simulink model "quantizedNetSim_4"  (R2025a)
settings: Solver=FixedStepAuto  StartTime=0.0  StopTime=10.0  RelTol=1e-3
undefined symbols (not defined in the file or in its folder): quantizedNet
libraries: dlconvfclib x9, dlactivationlib x3, dlpoolinglib x1, dlinputlayernormlib x1
settings Model: Creator=wenzheli  LastModifiedBy=wenzheli
settings OptimizationCC: DefaultParameterBehavior=Inlined  EnhancedBackFolding=on  PassReuseOutputArgsAs=Individual arguments  ZeroExternalMemoryAtStartup=off  ZeroInternalMemoryAtStartup=off  OptimizeBlockOrder=speed  DifferentSizesBufferReuse=on  OptimizationCustomize=off  EfficientTunableParamExpr=on
settings DebuggingCC: ParameterTunabilityLossMsg=error
settings SFSimCC: MATLABDynamicMemAlloc=off
settings RTWCC: SystemTargetFile=ert.tlc  TemplateMakefile=ert_default_tmf  Description=Embedded Coder
settings CodeAppCC: ForceParamTrailComments=on  IgnoreCustomStorageClasses=off  OperatorAnnotations=on  SimulinkDataObjDesc=on  SFDataObjDesc=on  InsertBlockDesc=on
settings ERTTargetCC: ExtModeTransport=0.0  ExtModeStaticAlloc=off  ExtModeMexFile=ext_comm  ExtModeIntrfLevel=Level1  ERTCustomFileTemplate=example_file_process.tlc  TargetLangStandard=C99 (ISO)  GenerateSampleERTMain=on

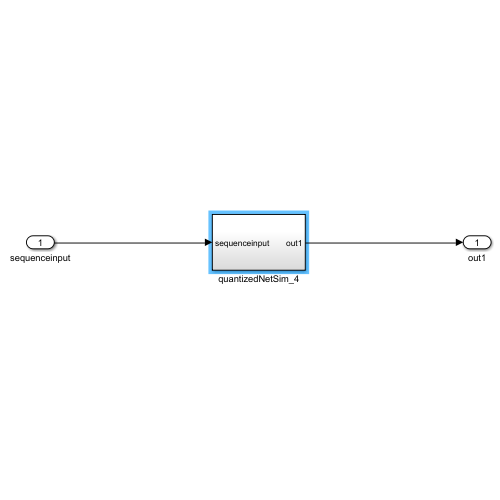
[thumbnail: Simulink's stored preview of the top-level diagram]
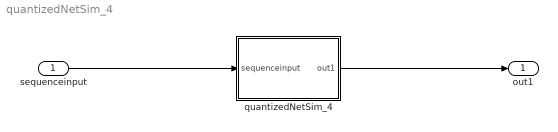
== system quantizedNetSim_4 ==
  sequenceinput : Inport  PortDimensions="[1  256]"
  quantizedNetSim_4 : Subsystem
  out1 : Outport
  wires:
  sequenceinput/1 -> quantizedNetSim_4/1(sequenceinput)
  quantizedNetSim_4/1(out1) -> out1/1

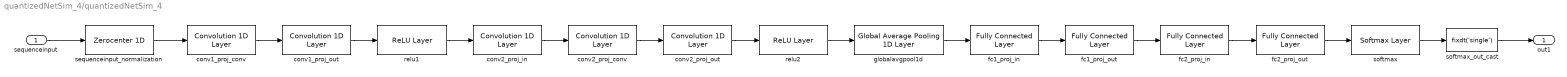
== system quantizedNetSim_4/quantizedNetSim_4 ==
  sequenceinput : Inport  PortDimensions="[1  256]"
  conv1_proj_conv : dlconvfclib/Convolution 1D Layer  Layer=quantizedNet.Layers(2)  PermuteDims=[2 1]  OutMin=[]  OutMax=[]  OutDataTypeStr=fixdt(1,8,1)  RndMeth=Nearest  SaturateOnIntegerOverflow=on  WeightsDataTypeStr=fixdt(1,8,7)  WeightsMin=[]  WeightsMax=[]  BiasDataTypeStr=fixdt(1,32,10)  BiasMin=[]  BiasMax=[]  AccumDataTypeStr=fixdt(1,32,10)  InternalRndMeth=Nearest  InternalSaturateOnIntegerOverflow=off  SampleTime=-1
      settings: DataFormat=CT
  conv1_proj_out : dlconvfclib/Convolution 1D Layer  Layer=quantizedNet.Layers(3)  PermuteDims=[2 1]  OutMin=[]  OutMax=[]  OutDataTypeStr=fixdt(1,8,2)  RndMeth=Nearest  SaturateOnIntegerOverflow=on  WeightsDataTypeStr=fixdt(1,8,7)  WeightsMin=[]  WeightsMax=[]  BiasDataTypeStr=fixdt(1,32,8)  BiasMin=[]  BiasMax=[]  AccumDataTypeStr=fixdt(1,32,8)  InternalRndMeth=Nearest  InternalSaturateOnIntegerOverflow=off  SampleTime=-1
      settings: DataFormat=CT
  conv2_proj_conv : dlconvfclib/Convolution 1D Layer  Layer=quantizedNet.Layers(6)  PermuteDims=[2 1]  OutMin=[]  OutMax=[]  OutDataTypeStr=fixdt(1,8,-2)  RndMeth=Nearest  SaturateOnIntegerOverflow=on  WeightsDataTypeStr=fixdt(1,8,7)  WeightsMin=[]  WeightsMax=[]  BiasDataTypeStr=fixdt(1,32,8)  BiasMin=[]  BiasMax=[]  AccumDataTypeStr=fixdt(1,32,8)  InternalRndMeth=Nearest  InternalSaturateOnIntegerOverflow=off  SampleTime=-1
      settings: DataFormat=CT
  conv2_proj_in : dlconvfclib/Convolution 1D Layer  Layer=quantizedNet.Layers(5)  PermuteDims=[2 1]  OutMin=[]  OutMax=[]  OutDataTypeStr=fixdt(1,8,1)  RndMeth=Nearest  SaturateOnIntegerOverflow=on  WeightsDataTypeStr=fixdt(1,8,7)  WeightsMin=[]  WeightsMax=[]  BiasDataTypeStr=fixdt(1,32,9)  BiasMin=[]  BiasMax=[]  AccumDataTypeStr=fixdt(1,32,9)  InternalRndMeth=Nearest  InternalSaturateOnIntegerOverflow=off  SampleTime=-1
      settings: DataFormat=CT
  conv2_proj_out : dlconvfclib/Convolution 1D Layer  Layer=quantizedNet.Layers(7)  PermuteDims=[2 1]  OutMin=[]  OutMax=[]  OutDataTypeStr=fixdt(1,8,-2)  RndMeth=Nearest  SaturateOnIntegerOverflow=on  WeightsDataTypeStr=fixdt(1,8,7)  WeightsMin=[]  WeightsMax=[]  BiasDataTypeStr=fixdt(1,32,5)  BiasMin=[]  BiasMax=[]  AccumDataTypeStr=fixdt(1,32,5)  InternalRndMeth=Nearest  InternalSaturateOnIntegerOverflow=off  SampleTime=-1
      settings: DataFormat=CT
  fc1_proj_in : dlconvfclib/Fully Connected Layer  Layer=quantizedNet.Layers(10)  OutMin=[]  OutMax=[]  OutDataTypeStr=fixdt(1,8,5)  RndMeth=Nearest  SaturateOnIntegerOverflow=on  WeightsDataTypeStr=fixdt(1,8,7)  WeightsMin=[]  WeightsMax=[]  BiasDataTypeStr=fixdt(1,32,10)  BiasMin=[]  BiasMax=[]  AccumDataTypeStr=fixdt(1,32,10)  AccumMin=[]  AccumMax=[]  InternalRndMeth=Nearest  InternalSaturateOnIntegerOverflow=off  SampleTime=-1
      settings: DataFormat=C
  fc1_proj_out : dlconvfclib/Fully Connected Layer  Layer=quantizedNet.Layers(11)  OutMin=[]  OutMax=[]  OutDataTypeStr=fixdt(1,8,6)  RndMeth=Nearest  SaturateOnIntegerOverflow=on  WeightsDataTypeStr=fixdt(1,8,7)  WeightsMin=[]  WeightsMax=[]  BiasDataTypeStr=fixdt(1,32,12)  BiasMin=[]  BiasMax=[]  AccumDataTypeStr=fixdt(1,32,12)  AccumMin=[]  AccumMax=[]  InternalRndMeth=Nearest  InternalSaturateOnIntegerOverflow=off  SampleTime=-1
      settings: DataFormat=C
  fc2_proj_in : dlconvfclib/Fully Connected Layer  Layer=quantizedNet.Layers(12)  OutMin=[]  OutMax=[]  OutDataTypeStr=fixdt(1,8,2)  RndMeth=Nearest  WeightsDataTypeStr=fixdt(1,8,7)  WeightsMin=[]  WeightsMax=[]  BiasDataTypeStr=fixdt(1,32,13)  BiasMin=[]  BiasMax=[]  AccumDataTypeStr=fixdt(1,32,13)  AccumMin=[]  AccumMax=[]  InternalRndMeth=Nearest  InternalSaturateOnIntegerOverflow=off  SampleTime=-1
      settings: DataFormat=C
  fc2_proj_out : dlconvfclib/Fully Connected Layer  Layer=quantizedNet.Layers(13)  OutMin=[]  OutMax=[]  OutDataTypeStr=fixdt(1,8,2)  RndMeth=Nearest  SaturateOnIntegerOverflow=on  WeightsDataTypeStr=fixdt(1,8,7)  WeightsMin=[]  WeightsMax=[]  BiasDataTypeStr=fixdt(1,32,9)  BiasMin=[]  BiasMax=[]  AccumDataTypeStr=fixdt(1,32,9)  AccumMin=[]  AccumMax=[]  InternalRndMeth=Nearest  InternalSaturateOnIntegerOverflow=off  SampleTime=-1
      settings: DataFormat=C
  globalavgpool1d : dlpoolinglib/Global Average Pooling 1D Layer  Layer=quantizedNet.Layers(9)  InputSize="[2  256]"  OutMin=[]  OutMax=[]  OutDataTypeStr=fixdt(1,8,3)  RndMeth=Nearest  SaturateOnIntegerOverflow=on  AccumDataTypeStr=fixdt(1,32,-2)  NumPoolingElementsDataTypeStr=fixdt(0,32,0)  NumPoolingElementsMin=[]  NumPoolingElementsMax=[]  InternalRndMeth=Nearest  InternalSaturateOnIntegerOverflow=on  SampleTime=-1
      settings: DataFormat=CT
  relu1 : dlactivationlib/ReLU Layer  OutMin=[]  OutMax=[]  OutDataTypeStr=fixdt(1,8,2)  SampleTime=-1
  relu2 : dlactivationlib/ReLU Layer  OutMin=[]  OutMax=[]  OutDataTypeStr=fixdt(1,8,-2)  SampleTime=-1
  sequenceinput_normalization : dlinputlayernormlib/Zerocenter 1D  Layer=quantizedNet.Layers(1)  OutMin=[]  OutMax=[]  OutDataTypeStr=fixdt(1,8,3)  RndMeth=Nearest  SaturateOnIntegerOverflow=on  MeanDataTypeStr=fixdt(0,8,13)  MeanMin=[]  MeanMax=[]  AccumDataTypeStr=fixdt(1,21,13)  InternalRndMeth=Nearest  InternalSaturateOnIntegerOverflow=on  SampleTime=-1
      settings: DataFormat=CT
  softmax : dlactivationlib/Softmax Layer  ApproximationMethod=Lookup  OutMin=[]  OutMax=[]  OutDataTypeStr=fixdt(0,8,8)  RndMeth=Nearest  SaturateOnIntegerOverflow=on  AccumDataTypeStr=fixdt(0,32,16)  InternalRndMeth=Nearest  InternalSaturateOnIntegerOverflow=on  SampleTime=-1
      settings: DataFormat=C
  softmax_out_cast : DataTypeConversion  OutDataTypeStr=fixdt('single')  RndMeth=Nearest
  out1 : Outport
  wires:
  conv1_proj_out/1 -> relu1/1
  conv1_proj_conv/1 -> conv1_proj_out/1
  sequenceinput_normalization/1 -> conv1_proj_conv/1
  softmax_out_cast/1 -> out1/1
  conv2_proj_conv/1 -> conv2_proj_out/1
  softmax/1 -> softmax_out_cast/1
  relu1/1 -> conv2_proj_in/1
  fc2_proj_out/1 -> softmax/1
  conv2_proj_out/1 -> relu2/1
  conv2_proj_in/1 -> conv2_proj_conv/1
  sequenceinput/1 -> sequenceinput_normalization/1
  fc1_proj_in/1 -> fc1_proj_out/1
  globalavgpool1d/1 -> fc1_proj_in/1
  fc1_proj_out/1 -> fc2_proj_in/1
  fc2_proj_in/1 -> fc2_proj_out/1
  relu2/1 -> globalavgpool1d/1
